simulink model "timeDelayedEKF_OOSM"  (R2015a)
settings: Solver=ode3  StartTime=0.0  StopTime=50  FixedStep=0.001  RelTol=1e-3
model workspace (MAT data in the model file):
  x_k = Simulink.Signal
  x_k.DataType = 'double'
  x_k.Dimensions = [2 1]
  x_k.DimensionsMode = 'Fixed'
  x_k.Complexity = 'real'
  x_k.SampleTime = -1
  x_k.SamplingMode = 'auto'
  x_k.InitialValue = '[0;0]'
  P_k = Simulink.Signal
  P_k.DataType = 'double'
  P_k.Dimensions = [2 2]
  P_k.DimensionsMode = 'Fixed'
  P_k.Complexity = 'real'
  P_k.SampleTime = -1
  P_k.SamplingMode = 'auto'
  P_k.InitialValue = '10*ones(2,2)'
  R = Simulink.Parameter
  R.Value = 0.001
  R.DataType = 'auto'
  t_delta = Simulink.Parameter
  t_delta.Value = 0.01
  t_delta.DataType = 'auto'
  x_d = Simulink.Signal
  x_d.DataType = 'auto'
  x_d.Dimensions = [2 1]
  x_d.DimensionsMode = 'auto'
  x_d.Complexity = 'auto'
  x_d.SampleTime = -1
  x_d.SamplingMode = 'auto'
  x_d.InitialValue = '[0;0]'
  P_d = Simulink.Signal
  P_d.DataType = 'auto'
  P_d.Dimensions = [2 2]
  P_d.DimensionsMode = 'auto'
  P_d.Complexity = 'auto'
  P_d.SampleTime = -1
  P_d.SamplingMode = 'auto'
  P_d.InitialValue = '10*eye(2,2)'
  U_n_d = Simulink.Signal
  U_n_d.DataType = 'auto'
  U_n_d.Dimensions = [2 2]
  U_n_d.DimensionsMode = 'auto'
  U_n_d.Complexity = 'auto'
  U_n_d.SampleTime = -1
  U_n_d.SamplingMode = 'auto'
  U_n_d.InitialValue = '10*eye(2,2)'
  FIFO_update_count = Simulink.Signal
  FIFO_update_count.DataType = 'auto'
  FIFO_update_count.Dimensions = -1
  FIFO_update_count.DimensionsMode = 'auto'
  FIFO_update_count.Complexity = 'auto'
  FIFO_update_count.SampleTime = -1
  FIFO_update_count.SamplingMode = 'auto'
  FIFO_update_count.InitialValue = '0'
  flag_OOSM_update = Simulink.Signal
  flag_OOSM_update.DataType = 'boolean'
  flag_OOSM_update.Dimensions = 1
  flag_OOSM_update.DimensionsMode = 'auto'
  flag_OOSM_update.Complexity = 'auto'
  flag_OOSM_update.SampleTime = -1
  flag_OOSM_update.SamplingMode = 'auto'
  flag_OOSM_update.InitialValue = 'false'
undefined symbols (not defined in the file): des, gcbh
libraries: simulink x5
settings Model: PauseTimes=0  NumberOfSteps=10  CovSFcnEnable=off  Creator=Iseberg  LastModifiedBy=Ana
settings DebuggingCC: SolverPrmCheckMsg=warning  MultiTaskDSMMsg=warning  MultiTaskCondExecSysMsg=warning  MultiTaskRateTransMsg=warning

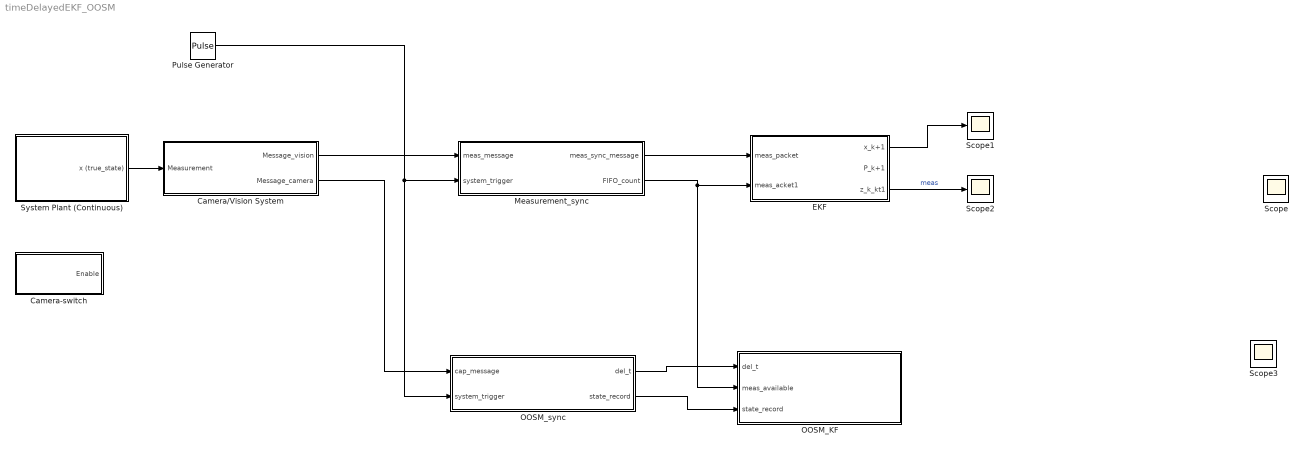
== system timeDelayedEKF_OOSM ==
  Camera-switch : Subsystem
  Camera/Vision System : Subsystem
  EKF : Subsystem
  Measurement_sync : Subsystem
  OOSM_KF : Subsystem
  OOSM_sync : Subsystem
  Pulse Generator : DiscretePulseGenerator  Period=10  SampleTime=0.001
  Scope{,1..3} (4 alike) : Scope
      Scope settings: YMin=0  YMax=1
      Scope1 settings: YMin=0  YMax=21000  SaveName=ScopeData12
      Scope2 settings: YMin=0  YMax=21000  SaveName=ScopeData3
      Scope3 settings: YMin=0  YMax=1  SaveName=ScopeData4
  System Plant (Continuous) : Subsystem
  wires:
  System Plant (Continuous)/1(x (true_state)) -> Camera/Vision System/1(Measurement)
  Camera/Vision System/1("Message_vision ") -> Measurement_sync/1(meas_message)
  Camera/Vision System/2("Message_camera ") -> OOSM_sync/1(cap_message)
  Pulse Generator/1 -> Measurement_sync/2("system_trigger "), OOSM_sync/2("system_trigger ")
  Measurement_sync/2(FIFO_count) -> EKF/2(meas_acket1), OOSM_KF/2(meas_available)
  OOSM_sync/1(del_t) -> OOSM_KF/1(del_t)
  Measurement_sync/1(meas_sync_message) -> EKF/1(meas_packet)
  EKF/3(z_k_kt1) -> Scope2/1  "meas"
  EKF/1(x_k+1) -> Scope1/1
  OOSM_sync/2(state_record) -> OOSM_KF/3("state_record ")

== system timeDelayedEKF_OOSM/Camera-switch ==
  Manual Switch : ManualSwitch
  Manual Switch1 : ManualSwitch  CurrentSetting=0
  Manual Switch2 : ManualSwitch
  Off_manual : Constant  Value=inf
  On_manual : Constant  Value=0.1
  Scope : Scope
      settings: SaveName=ScopeData6
  Step : Step  Time=abs(0.1*randn(1))  After=0.1  SampleTime=0
  intergeneration time : Constant  Value=0.1
  Enable : Outport
  wires:
  intergeneration time/1 -> Manual Switch/2
  Manual Switch2/1 -> Manual Switch1/1
  Off_manual/1 -> Manual Switch2/1
  Manual Switch1/1 -> Enable/1
  Step/1 -> Scope/1, Manual Switch/1
  Manual Switch/1 -> Manual Switch1/2
  On_manual/1 -> Manual Switch2/2

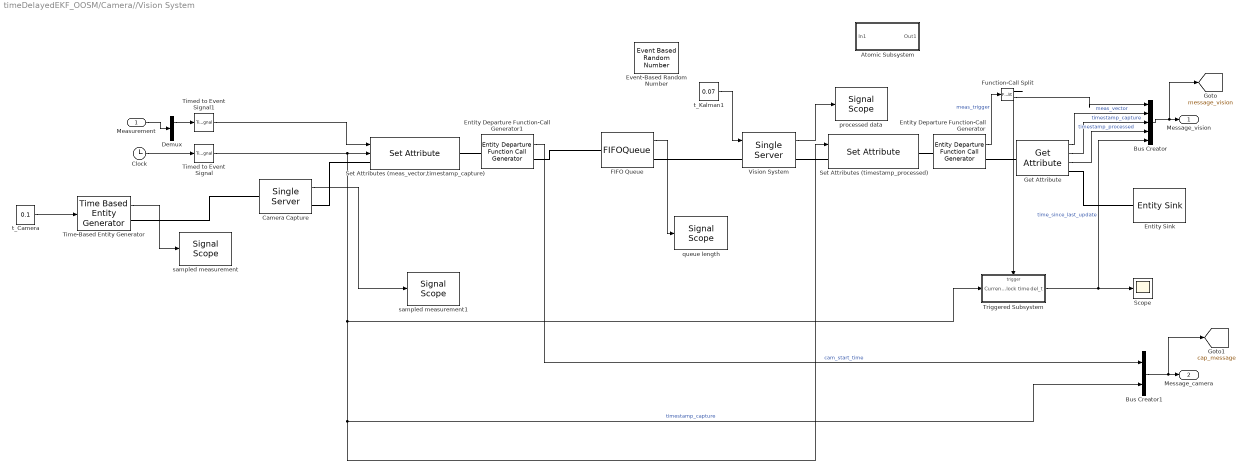
== system timeDelayedEKF_OOSM/Camera//Vision System ==
  Measurement : Inport
  Atomic Subsystem : Subsystem
  Bus Creator : BusCreator  Inputs=5
  Bus Creator1 : BusCreator  Inputs=2
  Camera Capture : SingleServer  ServiceTime=0  StatNumberDeparted=on
  Clock : Clock
      settings: Decimation=2
  Demux : Demux  Outputs=2
  Entity Departure Function-Call Generator : EntityDepartureFunctionCallGenerator
  Entity Departure Function-Call Generator1 : EntityDepartureFunctionCallGenerator  TimingFunctionCallF1=Before entity departure
  Entity Sink : EntitySink
  Event-Based Random Number : EventBasedRandomNumber  Distribution=Uniform  minUnif=0.05  maxUnif=0.08
  FIFO Queue : FIFOQueue  Capacity=1  StatNumberInBlock=on
      settings: OutputPortMap=o1
  Function-Call Split : FunctionCallSplit
  Get Attribute : GetAttribute  AttributeName=meas_vector|timestamp_capture|timestamp_processed  AttributeMissing=Error|Error|Error  AttributeDefaultValue=1|1|1  AttributeTreatAsVector=1|1|1  AttributeSendTiming=After entity departure|After entity departure|After entity departure  EvaluatedDefaultAttributeValue={ [];[];[]}
      settings: OutputPortMap=o1,o2,o3
  Scope : Scope
  Set Attributes (meas_vector,timestamp_capture) : SetAttribute  AttributeName=meas_vector|timestamp_capture  AttributeFrom=Signal port|Signal port  AttributeValue=1|1  AttributeTreatAsVector=1|1  EvaluatedAttributeValue={ [];[]}
      settings: InputPortMap=u0,u1
  Set Attributes (timestamp_processed) : SetAttribute  AttributeName=timestamp_processed  AttributeFrom=Signal port  EvaluatedAttributeValue={ []}
  Time-Based Entity Generator : TimeBasedEntityGenerator  GenerateEntitiesUpon=Intergeneration time from port t  StatNumberDeparted=on
  Timed to Event Signal : TimedToEventSignal
  Timed to Event Signal1 : TimedToEventSignal
  Triggered Subsystem : Subsystem  TreatAsAtomicUnit=on
  "Vision System " : SingleServer  ServiceTimeFrom=Signal port t  StatNumberDeparted=on
  processed data : SignalScope  LoadFcn=des.scope.CallbackSupport('seLoadFcn',gcbh)  StartFcn=des.scope.CallbackSupport('seStartFcn',gcbh)  StopFcn=des.scope.CallbackSupport('seStopFcn',gcbh)
      settings: CopyFcn=des.scope.CallbackSupport('seCopyFcn',gcbh)  DeleteFcn=des.scope.CallbackSupport('seDeleteFcn',gcbh)  PreSaveFcn=des.scope.CallbackSupport('sePreSaveFcn',gcbh)  NameChangeFcn=des.scope.CallbackSupport('seNameChangeFcn',gcbh)  OpenFcn=des.scope.CallbackSupport('seOpenFcn',gcbh)
  queue length : SignalScope  LoadFcn=des.scope.CallbackSupport('seLoadFcn',gcbh)  StartFcn=des.scope.CallbackSupport('seStartFcn',gcbh)  StopFcn=des.scope.CallbackSupport('seStopFcn',gcbh)
      settings: CopyFcn=des.scope.CallbackSupport('seCopyFcn',gcbh)  DeleteFcn=des.scope.CallbackSupport('seDeleteFcn',gcbh)  PreSaveFcn=des.scope.CallbackSupport('sePreSaveFcn',gcbh)  NameChangeFcn=des.scope.CallbackSupport('seNameChangeFcn',gcbh)  OpenFcn=des.scope.CallbackSupport('seOpenFcn',gcbh)
  sampled measurement : SignalScope  LoadFcn=des.scope.CallbackSupport('seLoadFcn',gcbh)  StartFcn=des.scope.CallbackSupport('seStartFcn',gcbh)  StopFcn=des.scope.CallbackSupport('seStopFcn',gcbh)
      settings: CopyFcn=des.scope.CallbackSupport('seCopyFcn',gcbh)  DeleteFcn=des.scope.CallbackSupport('seDeleteFcn',gcbh)  PreSaveFcn=des.scope.CallbackSupport('sePreSaveFcn',gcbh)  NameChangeFcn=des.scope.CallbackSupport('seNameChangeFcn',gcbh)  OpenFcn=des.scope.CallbackSupport('seOpenFcn',gcbh)
  sampled measurement1 : SignalScope  LoadFcn=des.scope.CallbackSupport('seLoadFcn',gcbh)  StartFcn=des.scope.CallbackSupport('seStartFcn',gcbh)  StopFcn=des.scope.CallbackSupport('seStopFcn',gcbh)
      settings: CopyFcn=des.scope.CallbackSupport('seCopyFcn',gcbh)  DeleteFcn=des.scope.CallbackSupport('seDeleteFcn',gcbh)  PreSaveFcn=des.scope.CallbackSupport('sePreSaveFcn',gcbh)  NameChangeFcn=des.scope.CallbackSupport('seNameChangeFcn',gcbh)  OpenFcn=des.scope.CallbackSupport('seOpenFcn',gcbh)
  t_Camera : Constant  Value=0.1
  t_Kalman1 : Constant  Value=0.07
  "Message_vision " : Outport
  "Message_camera " : Outport  Port=2
  tag scope: cap_message=global, message_vision=global
  wires:
  Timed to Event Signal1/1 -> Set Attributes (meas_vector,timestamp_capture)/1
  Timed to Event Signal/1 -> Triggered Subsystem/1(Current Clock time), Bus Creator1/2, Set Attributes (timestamp_processed)/1, Set Attributes (meas_vector,timestamp_capture)/2  "timestamp_capture"
  Get Attribute/3 -> Bus Creator/4  "timestamp_processed"
  Time-Based Entity Generator/1 -> sampled measurement/1
  FIFO Queue/1 -> queue length/1
  "Vision System "/1 -> processed data/1
  Entity Departure Function-Call Generator/1 -> Function-Call Split/1  "meas_trigger"
  Get Attribute/2 -> Bus Creator/3  "timestamp_capture"
  Get Attribute/1 -> Bus Creator/2  "meas_vector"
  Clock/1 -> Timed to Event Signal/1
  Triggered Subsystem/1(del_t) -> Bus Creator/5, Scope/1  "time_since_last_update"
  Bus Creator1/1 -> [cap_message], "Message_camera "/1
  Entity Departure Function-Call Generator1/1 -> Bus Creator1/1  "cam_start_time"
  t_Camera/1 -> Time-Based Entity Generator/1
  Camera Capture/1 -> sampled measurement1/1
  Function-Call Split/2 -> Bus Creator/1
  Function-Call Split/1 -> Triggered Subsystem/Trigger
  Measurement/1 -> Demux/1
  Demux/1 -> Timed to Event Signal1/1
  t_Kalman1/1 -> "Vision System "/1
  Bus Creator/1 -> [message_vision], "Message_vision "/1
  connections:
  Entity Departure Function-Call Generator/LConn1 -- Set Attributes (timestamp_processed)/RConn1
  Get Attribute/RConn1 -- Entity Sink/LConn1
  "Vision System "/RConn1 -- Set Attributes (timestamp_processed)/LConn1
  Get Attribute/LConn1 -- Entity Departure Function-Call Generator/RConn1
  Entity Departure Function-Call Generator1/RConn1 -- FIFO Queue/LConn1
  Set Attributes (meas_vector,timestamp_capture)/RConn1 -- Entity Departure Function-Call Generator1/LConn1
  FIFO Queue/RConn1 -- "Vision System "/LConn1
  Camera Capture/LConn1 -- Time-Based Entity Generator/RConn1
  Camera Capture/RConn1 -- Set Attributes (meas_vector,timestamp_capture)/LConn1

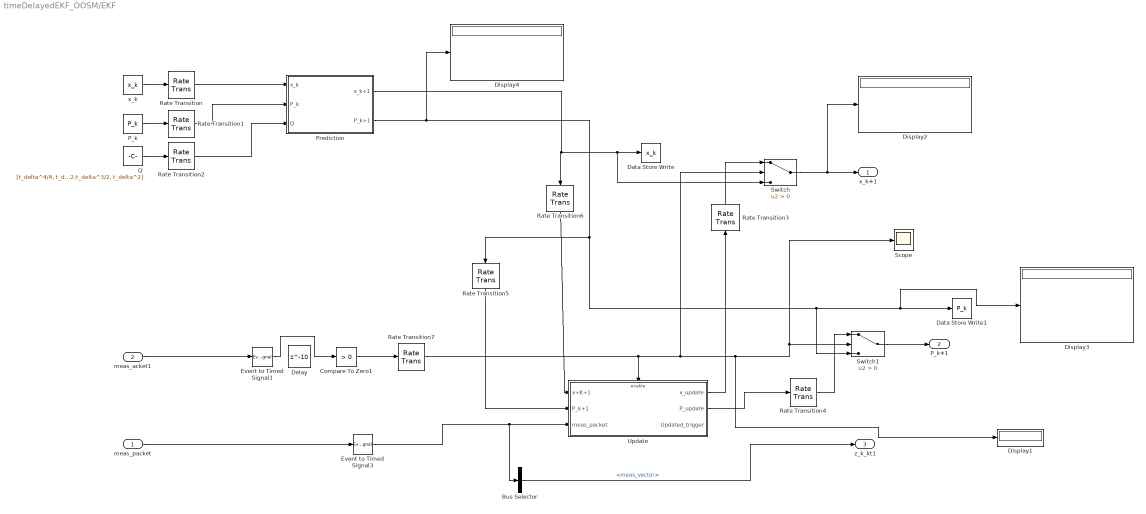
== system timeDelayedEKF_OOSM/EKF ==
  meas_packet : Inport
  meas_acket1 : Inport  Port=2
  Bus Selector : BusSelector  OutputSignals=meas_vector
  Compare To Zero1 : simulink/Logic and Bit Operations/Compare To Zero  relop=>  OutDataTypeStr=boolean
  Data Store Write : DataStoreWrite  DataStoreName=x_k  DataStoreElements=x_k
  Data Store Write1 : DataStoreWrite  DataStoreName=P_k  DataStoreElements=P_k
  Delay : Delay  DelayLength=10  InitialCondition=0
  Display{1..4} (4 alike) : Display
  Event to Timed Signal1 : EventToTimedSignal
  Event to Timed Signal3 : EventToTimedSignal
  P_k : DataStoreRead  DataStoreName=P_k  DataStoreElements=P_k
  Prediction : Subsystem  TreatAsAtomicUnit=on  SystemSampleTime=0.01
  Q : Constant  Value=[t_delta^4/4, t_delta^3/2;t_delta^3/2, t_delta^2]
  Rate Transition{,1..6} (7 alike) : RateTransition
  Rate Transition7 : RateTransition  OutPortSampleTime=0.01
  Scope : Scope
      settings: SaveName=ScopeData9
  Switch : Switch  Criteria=u2 > Threshold
  Switch1 : Switch  Criteria=u2 > Threshold
  Update : Subsystem  TreatAsAtomicUnit=on
  x_k : DataStoreRead  DataStoreName=x_k  DataStoreElements=x_k
  x_k+1 : Outport
  "P_k+1 " : Outport  Port=2
  z_k_kt1 : Outport  Port=3
  wires:
  x_k/1 -> Rate Transition/1
  P_k/1 -> Rate Transition1/1
  Q/1 -> Rate Transition2/1
  Prediction/1(x_k+1) -> Switch/3, Data Store Write/1, Rate Transition6/1
  Switch/1 -> Display2/1, x_k+1/1
  Switch1/1 -> "P_k+1 "/1
  Rate Transition/1 -> Prediction/1(x_k)
  Rate Transition1/1 -> Prediction/2(P_k)
  Rate Transition2/1 -> Prediction/3(Q)
  Prediction/2(P_k+1) -> Display4/1, Switch1/3, Display3/1, Data Store Write1/1, Rate Transition5/1
  Rate Transition6/1 -> Update/1(x+K+1)
  Rate Transition5/1 -> Update/2(P_k+1)
  Update/1(x_update) -> Rate Transition3/1
  Rate Transition4/1 -> Switch1/1
  Rate Transition3/1 -> Switch/1
  Update/2(P_update) -> Rate Transition4/1
  meas_packet/1 -> Event to Timed Signal3/1
  meas_acket1/1 -> Event to Timed Signal1/1
  Event to Timed Signal3/1 -> Bus Selector/1, Update/3(meas_packet)
  Rate Transition7/1 -> Switch/2, Display1/1, Scope/1, Switch1/2, Update/Enable
  Compare To Zero1/1 -> Rate Transition7/1
  Event to Timed Signal1/1 -> Compare To Zero1/1
  Bus Selector/1 -> z_k_kt1/1  "<meas_vector>"

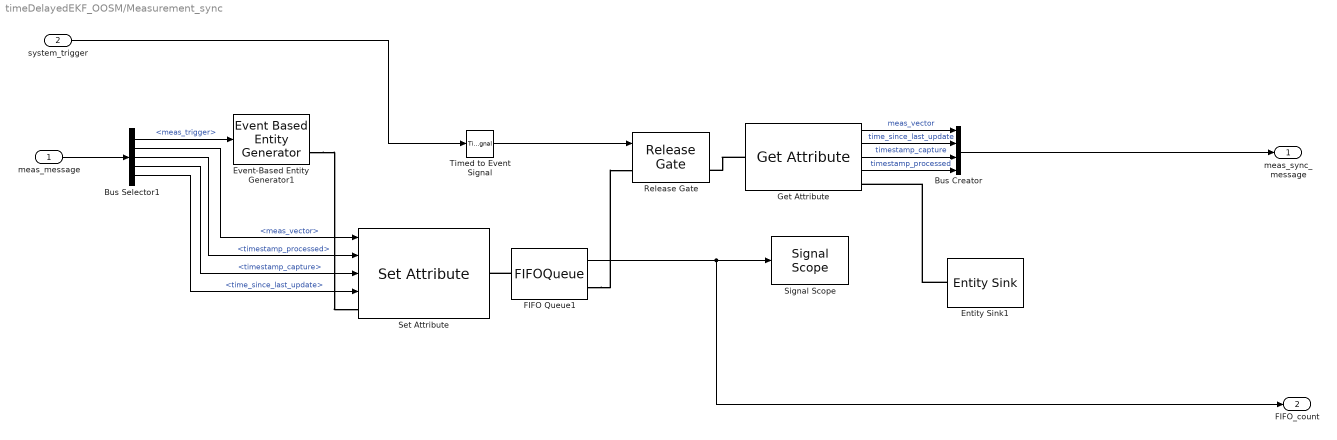
== system timeDelayedEKF_OOSM/Measurement_sync ==
  meas_message : Inport
  "system_trigger " : Inport  Port=2
  Bus Creator : BusCreator
  Bus Selector1 : BusSelector  OutputSignals=meas_trigger,meas_vector,timestamp_processed,timestamp_capture,time_since_last_update
  Entity Sink1 : EntitySink
  Event-Based Entity Generator1 : EventBasedEntityGenerator  GenerateEntitiesUpon=Function call from port fcn  StatNumberDeparted=on
  FIFO Queue1 : FIFOQueue  Capacity=1  StatNumberInBlock=on
      settings: OutputPortMap=o1
  Get Attribute : GetAttribute  AttributeName=meas_vector|time_since_last_update|timestamp_capture|timestamp_processed  AttributeMissing=Error|Error|Error|Error  AttributeDefaultValue=1|1|1|1  AttributeTreatAsVector=1|1|1|1  AttributeSendTiming=After entity departure|After entity departure|After entity departure|After entity departure  EvaluatedDefaultAttributeValue={ [];[];[];[]}
      settings: OutputPortMap=o1,o2,o3,o4
  Release Gate : ReleaseGate  StatNumberDeparted=on
  Set Attribute : SetAttribute  AttributeName=meas_vector|timestamp_processed|timestamp_capture|time_since_last_update  AttributeFrom=Signal port|Signal port|Signal port|Signal port  AttributeValue=1|1|1|1  AttributeTreatAsVector=1|1|1|1  EvaluatedAttributeValue={ [];[];[];[]}
      settings: InputPortMap=u0,u1,u2,u3
  Signal Scope : SignalScope  LoadFcn=des.scope.CallbackSupport('seLoadFcn',gcbh)  StartFcn=des.scope.CallbackSupport('seStartFcn',gcbh)  StopFcn=des.scope.CallbackSupport('seStopFcn',gcbh)
      settings: CopyFcn=des.scope.CallbackSupport('seCopyFcn',gcbh)  DeleteFcn=des.scope.CallbackSupport('seDeleteFcn',gcbh)  PreSaveFcn=des.scope.CallbackSupport('sePreSaveFcn',gcbh)  NameChangeFcn=des.scope.CallbackSupport('seNameChangeFcn',gcbh)  OpenFcn=des.scope.CallbackSupport('seOpenFcn',gcbh)
  Timed to Event Signal : TimedToEventSignal
  meas_sync_message : Outport
  FIFO_count : Outport  Port=2
  wires:
  Get Attribute/4 -> Bus Creator/4  "timestamp_processed"
  Bus Selector1/1 -> Event-Based Entity Generator1/1  "<meas_trigger>"
  Get Attribute/3 -> Bus Creator/3  "timestamp_capture"
  Bus Selector1/2 -> Set Attribute/1  "<meas_vector>"
  Get Attribute/2 -> Bus Creator/2  "time_since_last_update"
  "system_trigger "/1 -> Timed to Event Signal/1
  Get Attribute/1 -> Bus Creator/1  "meas_vector"
  Bus Selector1/5 -> Set Attribute/4  "<time_since_last_update>"
  Bus Selector1/3 -> Set Attribute/2  "<timestamp_processed>"
  Bus Selector1/4 -> Set Attribute/3  "<timestamp_capture>"
  Timed to Event Signal/1 -> Release Gate/1
  meas_message/1 -> Bus Selector1/1
  Bus Creator/1 -> meas_sync_message/1
  FIFO Queue1/1 -> FIFO_count/1, Signal Scope/1
  connections:
  Entity Sink1/LConn1 -- Get Attribute/RConn1
  FIFO Queue1/RConn1 -- Release Gate/LConn1
  Event-Based Entity Generator1/RConn1 -- Set Attribute/LConn1
  Get Attribute/LConn1 -- Release Gate/RConn1
  FIFO Queue1/LConn1 -- Set Attribute/RConn1

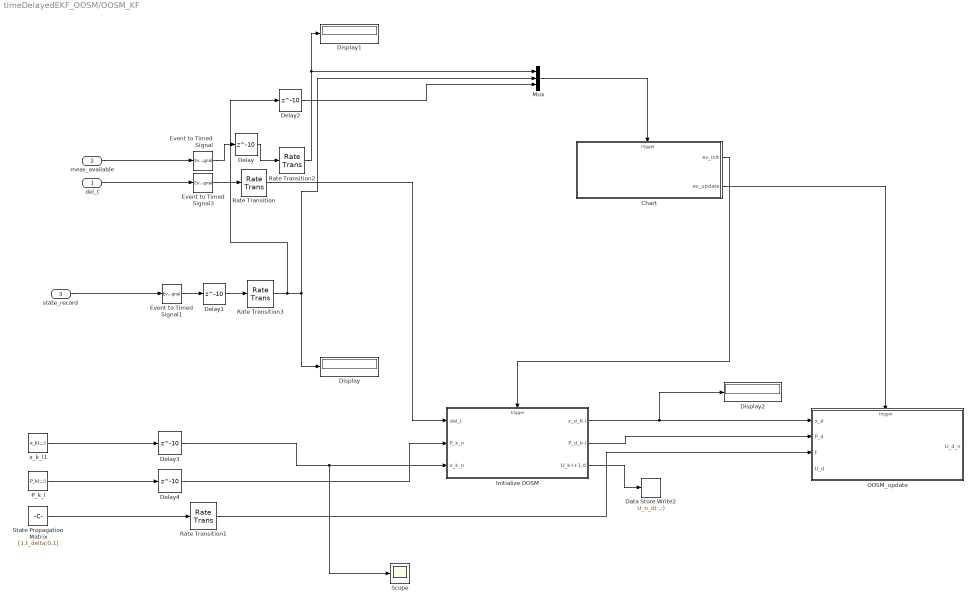
== system timeDelayedEKF_OOSM/OOSM_KF ==
  del_t : Inport
  meas_available : Inport  Port=2
  "state_record " : Inport  Port=3
  Chart : Stateflow chart  TreatAsAtomicUnit=on
  Data Store Write2 : DataStoreWrite  DataStoreName=U_n_d  DataStoreElements=U_n_d(:,:)
  Delay : Delay  DelayLength=10  InitialCondition=0
  Delay1 : Delay  DelayLength=10  InitialCondition=0
  Delay2 : Delay  DelayLength=10  InitialCondition=0
  Delay3 : Delay  DelayLength=10  InitialCondition=0  SampleTime=0.01
  Delay4 : Delay  DelayLength=10  InitialCondition=10  SampleTime=0.01
  Display : Display
  Display1 : Display
  Display2 : Display
  Event to Timed Signal : EventToTimedSignal
  Event to Timed Signal1 : EventToTimedSignal
  Event to Timed Signal3 : EventToTimedSignal
  Initialize OOSM : Subsystem  TreatAsAtomicUnit=on
  Mux : Mux  Inputs=3
  OOSM_update : Subsystem
  P_k_l : DataStoreRead  DataStoreName=P_k  DataStoreElements=P_k(:,:)
  Rate Transition{,1..3} (4 alike) : RateTransition
  Scope : Scope
      settings: SaveName=ScopeData14
  "State Propagation Matrix " : Constant  Value=[1,t_delta;0,1]
  x_k_l1 : DataStoreRead  DataStoreName=x_k  DataStoreElements=x_k(:,:)
  wires:
  "State Propagation Matrix "/1 -> Rate Transition1/1
  del_t/1 -> Event to Timed Signal3/1
  Event to Timed Signal3/1 -> Rate Transition/1
  meas_available/1 -> Event to Timed Signal/1
  Event to Timed Signal1/1 -> Delay1/1
  Delay1/1 -> Rate Transition3/1
  "state_record "/1 -> Event to Timed Signal1/1
  Rate Transition3/1 -> Delay2/1, Mux/2, Display/1
  Event to Timed Signal/1 -> Delay/1
  Rate Transition2/1 -> Mux/1, Display1/1
  P_k_l/1 -> Delay4/1
  x_k_l1/1 -> Delay3/1
  Delay4/1 -> Initialize OOSM/2(P_k_n)
  Delay3/1 -> Scope/1, Initialize OOSM/3(x_k_n)
  Rate Transition/1 -> Initialize OOSM/1(del_t)
  Initialize OOSM/1(x_d_K-l) -> Display2/1, OOSM_update/1(x_d)
  Initialize OOSM/2(P_d_k-l) -> OOSM_update/2(P_d)
  Rate Transition1/1 -> OOSM_update/3(F)
  Mux/1 -> Chart/Trigger
  Chart/1(ev_init) -> Initialize OOSM/Trigger
  Chart/2(ev_update) -> OOSM_update/Trigger
  Delay/1 -> Rate Transition2/1
  Delay2/1 -> Mux/3
  Initialize OOSM/3(U_k-l+1,d) -> Data Store Write2/1

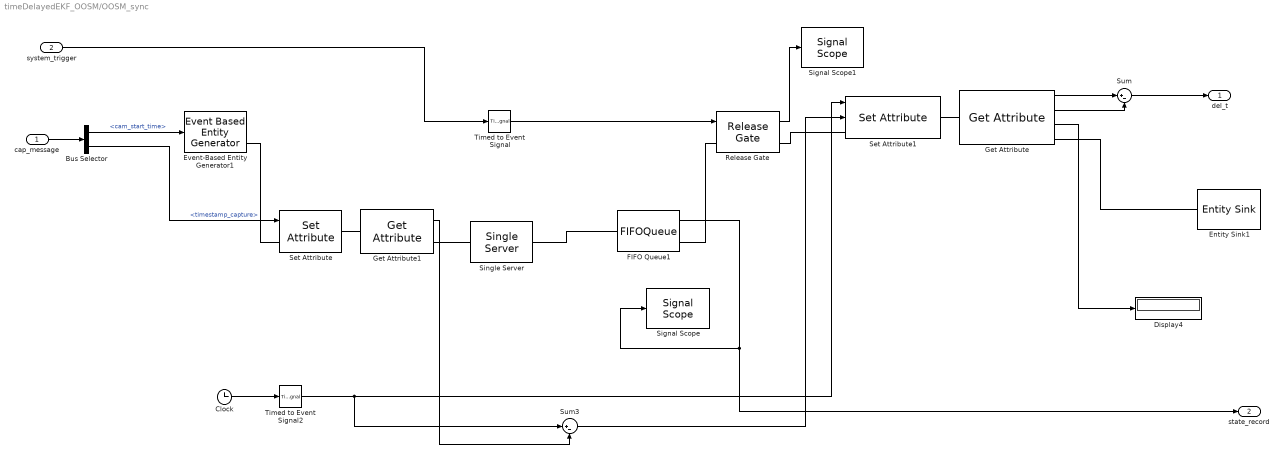
== system timeDelayedEKF_OOSM/OOSM_sync ==
  cap_message : Inport
  "system_trigger " : Inport  Port=2
  Bus Selector : BusSelector  OutputSignals=cam_start_time,timestamp_capture
  Clock : Clock
  Display4 : Display
  Entity Sink1 : EntitySink
  Event-Based Entity Generator1 : EventBasedEntityGenerator  GenerateEntitiesUpon=Function call from port fcn  StatNumberDeparted=on
  FIFO Queue1 : FIFOQueue  Capacity=5  StatNumberInBlock=on
      settings: OutputPortMap=o1
  Get Attribute : GetAttribute  AttributeName=timestamp_KFTrigger|timestamp_capture|t_delta_oosm  AttributeMissing=Error|Error|Error  AttributeDefaultValue=1|1|1  AttributeTreatAsVector=1|1|1  AttributeSendTiming=After entity departure|After entity departure|After entity departure  EvaluatedDefaultAttributeValue={ [];[];[]}
      settings: OutputPortMap=o1,o2,o3
  Get Attribute1 : GetAttribute  AttributeName=timestamp_capture  EvaluatedDefaultAttributeValue={ []}
      settings: OutputPortMap=o1
  Release Gate : ReleaseGate  StatNumberDeparted=on
  Set Attribute : SetAttribute  AttributeName=timestamp_capture  AttributeFrom=Signal port  EvaluatedAttributeValue={ []}
  Set Attribute1 : SetAttribute  AttributeName=timestamp_KFTrigger|t_delta_oosm  AttributeFrom=Signal port|Signal port  AttributeValue=1|1  AttributeTreatAsVector=1|1  EvaluatedAttributeValue={ [];[]}
      settings: InputPortMap=u0,u1
  Signal Scope : SignalScope  LoadFcn=des.scope.CallbackSupport('seLoadFcn',gcbh)  StartFcn=des.scope.CallbackSupport('seStartFcn',gcbh)  StopFcn=des.scope.CallbackSupport('seStopFcn',gcbh)
      settings: CopyFcn=des.scope.CallbackSupport('seCopyFcn',gcbh)  DeleteFcn=des.scope.CallbackSupport('seDeleteFcn',gcbh)  PreSaveFcn=des.scope.CallbackSupport('sePreSaveFcn',gcbh)  NameChangeFcn=des.scope.CallbackSupport('seNameChangeFcn',gcbh)  OpenFcn=des.scope.CallbackSupport('seOpenFcn',gcbh)
  Signal Scope1 : SignalScope  LoadFcn=des.scope.CallbackSupport('seLoadFcn',gcbh)  StartFcn=des.scope.CallbackSupport('seStartFcn',gcbh)  StopFcn=des.scope.CallbackSupport('seStopFcn',gcbh)
      settings: CopyFcn=des.scope.CallbackSupport('seCopyFcn',gcbh)  DeleteFcn=des.scope.CallbackSupport('seDeleteFcn',gcbh)  PreSaveFcn=des.scope.CallbackSupport('sePreSaveFcn',gcbh)  NameChangeFcn=des.scope.CallbackSupport('seNameChangeFcn',gcbh)  OpenFcn=des.scope.CallbackSupport('seOpenFcn',gcbh)
  Single Server : SingleServer  ServiceTime=0
  Sum : Sum  Inputs=|+-
  Sum3 : Sum  Inputs=|+-
  Timed to Event Signal : TimedToEventSignal
  Timed to Event Signal2 : TimedToEventSignal
  del_t : Outport
  state_record : Outport  Port=2
  wires:
  FIFO Queue1/1 -> state_record/1, Signal Scope/1
  Bus Selector/1 -> Event-Based Entity Generator1/1  "<cam_start_time>"
  Bus Selector/2 -> Set Attribute/1  "<timestamp_capture>"
  Clock/1 -> Timed to Event Signal2/1
  Timed to Event Signal2/1 -> Sum3/1, Set Attribute1/1
  Get Attribute/1 -> Sum/1
  Get Attribute/2 -> Sum/2
  Get Attribute1/1 -> Sum3/2
  Sum3/1 -> Set Attribute1/2
  cap_message/1 -> Bus Selector/1
  "system_trigger "/1 -> Timed to Event Signal/1
  Timed to Event Signal/1 -> Release Gate/1
  Get Attribute/3 -> Display4/1
  Release Gate/1 -> Signal Scope1/1
  Sum/1 -> del_t/1
  connections:
  Event-Based Entity Generator1/RConn1 -- Set Attribute/LConn1
  FIFO Queue1/RConn1 -- Release Gate/LConn1
  Release Gate/RConn1 -- Set Attribute1/LConn1
  Set Attribute1/RConn1 -- Get Attribute/LConn1
  Get Attribute1/LConn1 -- Set Attribute/RConn1
  Single Server/RConn1 -- FIFO Queue1/LConn1
  Get Attribute1/RConn1 -- Single Server/LConn1
  Entity Sink1/LConn1 -- Get Attribute/RConn1

== system timeDelayedEKF_OOSM/System Plant (Continuous) ==
  Integrator : Integrator  InitialConditionSource=external
  Product1 : Product  Multiplication=Matrix(*)
  State Matrix 1 : Constant  Value=[5;1]
  State Matrix 2 : Constant  Value=[0,1;0,0]
  x (true_state) : Outport
  wires:
  State Matrix 1/1 -> Integrator/2
  State Matrix 2/1 -> Product1/1
  Integrator/1 -> x (true_state)/1, Product1/2
  Product1/1 -> Integrator/1

== system timeDelayedEKF_OOSM/Camera//Vision System/Atomic Subsystem ==
  In1 : Inport
  Constant : Constant  Value=100
  Gain : Gain  Gain=100
  Product : Product
  Rounding Function : Rounding
  Scope : Scope
      settings: SaveName=ScopeData5
  Out1 : Outport
  wires:
  In1/1 -> Gain/1
  Gain/1 -> Rounding Function/1
  Constant/1 -> Product/2
  Product/1 -> Scope/1, Out1/1
  Rounding Function/1 -> Product/1

== system timeDelayedEKF_OOSM/Camera//Vision System/Triggered Subsystem ==
  Current Clock time : Inport
  Trigger : TriggerPort  TriggerType=function-call
  Delay : Delay  DelayLength=1  InitialCondition=0
  Sum : Sum  Inputs=|+-
  del_t : Outport
  wires:
  Current Clock time/1 -> Sum/1, Delay/1
  Sum/1 -> del_t/1
  Delay/1 -> Sum/2

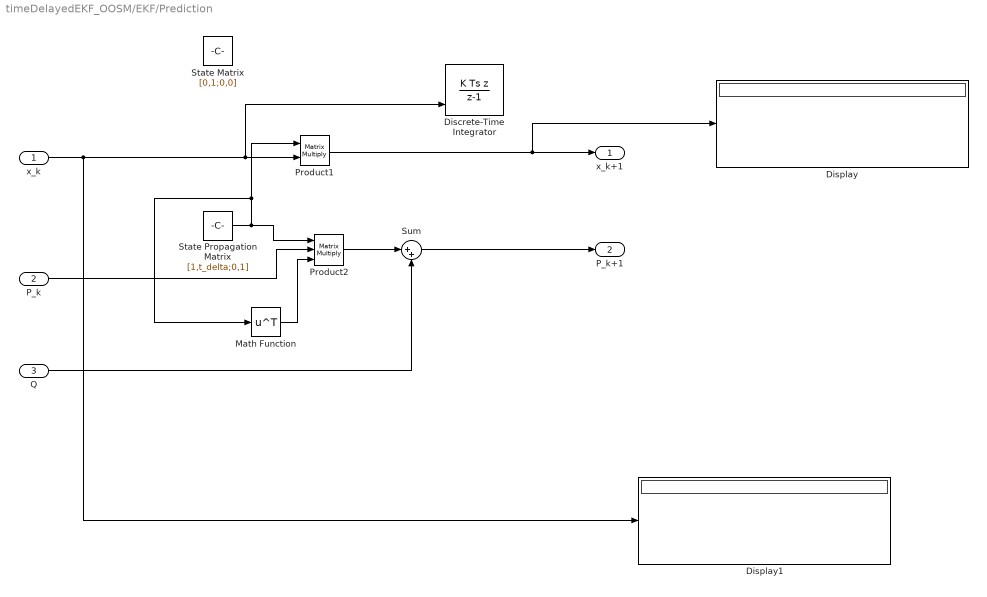
== system timeDelayedEKF_OOSM/EKF/Prediction ==
  x_k : Inport
  P_k : Inport  Port=2
  Q : Inport  Port=3
  Discrete-Time Integrator : DiscreteIntegrator  IntegratorMethod=Integration: Backward Euler  ExternalReset=rising  InitialConditionSource=external  InitialCondition=x_k  SampleTime=-1
  Display : Display
  Display1 : Display
  Math Function : Math  Operator=transpose  SaturateOnIntegerOverflow=on
  Product1 : Product  Multiplication=Matrix(*)
  Product2 : Product  Inputs=3  Multiplication=Matrix(*)
  State Matrix : Constant  Value=[0,1;0,0]
  "State Propagation Matrix " : Constant  Value=[1,t_delta;0,1]
  Sum : Sum  Inputs=|++
  x_k+1 : Outport
  P_k+1 : Outport  Port=2
  wires:
  Product2/1 -> Sum/1
  Q/1 -> Sum/2
  P_k/1 -> Product2/2
  Sum/1 -> P_k+1/1
  "State Propagation Matrix "/1 -> Product1/1, Math Function/1, Product2/1
  Math Function/1 -> Product2/3
  x_k/1 -> Display1/1, Discrete-Time Integrator/3, Product1/2
  Product1/1 -> Display/1, x_k+1/1

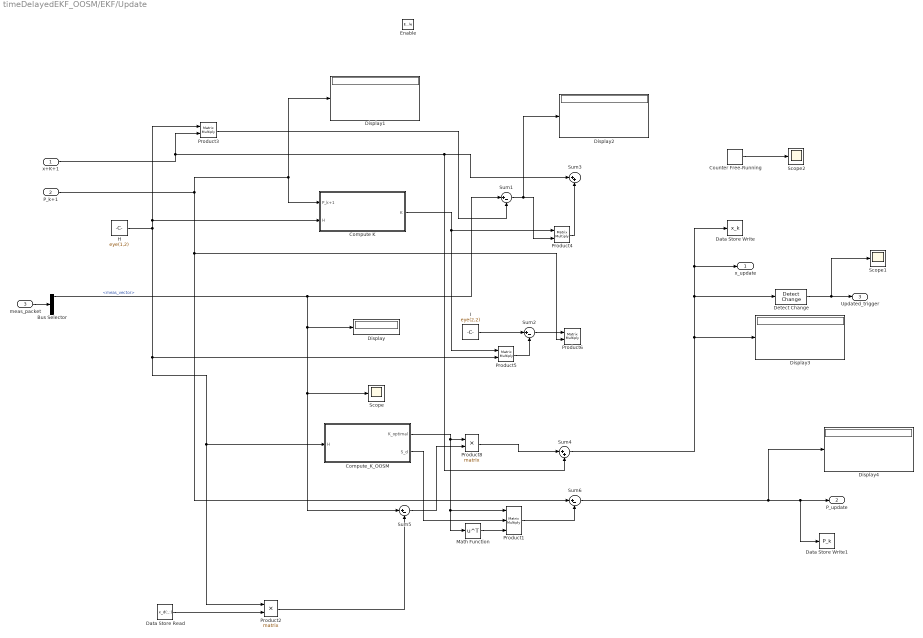
== system timeDelayedEKF_OOSM/EKF/Update ==
  x+K+1 : Inport
  P_k+1 : Inport  Port=2
  meas_packet : Inport  Port=3
  Enable : EnablePort
  Bus Selector : BusSelector  OutputSignals=meas_vector,time_since_last_update,timestamp_capture,timestamp_processed
  Compute K : Subsystem
  Compute_K_OOSM : Subsystem
  Counter Free-Running : simulink/Sources/Counter Free-Running  NumBits=16  tsamp=-1
  Data Store Read : DataStoreRead  DataStoreName=x_d  DataStoreElements=x_d(:,:)
  Data Store Write : DataStoreWrite  DataStoreName=x_k
  Data Store Write1 : DataStoreWrite  DataStoreName=P_k
  Detect Change : simulink/Logic and Bit Operations/Detect Change  vinit=0  InputProcessing=Inherited  OutDataTypeStr=boolean
  Display{,1..4} (5 alike) : Display
  H : Constant  Value=eye(1,2)  VectorParams1D=off
  I : Constant  Value=eye(2,2)
  Math Function : Math  Operator=transpose  SaturateOnIntegerOverflow=on
  Product1 : Product  Inputs=3  Multiplication=Matrix(*)
  Product{2..6,8} (6 alike) : Product  Multiplication=Matrix(*)
  Scope : Scope
      settings: TimeRange=5  SaveName=ScopeData11
  Scope1 : Scope
      settings: TimeRange=5  SaveName=ScopeData7
  Scope2 : Scope
      settings: TimeRange=50  YMin=0  YMax=4  SaveName=ScopeData8
  Sum{1..2,5..6} (4 alike) : Sum  Inputs=|+-
  Sum3 : Sum  Inputs=|++
  Sum4 : Sum  Inputs=|++
  x_update : Outport
  P_update : Outport  Port=2
  Updated_trigger : Outport  Port=3
  wires:
  P_k+1/1 -> Compute K/1(P_k+1), Display1/1, Sum6/1, Product6/2
  H/1 -> Compute K/2(H), Product3/1, Product2/1, Compute_K_OOSM/1(H), Product5/2
  x+K+1/1 -> Sum4/2, Sum3/1, Product3/2
  Bus Selector/1 -> Sum1/1, Display/1, Scope/1, Sum5/1  "<meas_vector>"
  Product3/1 -> Sum1/2
  Sum1/1 -> Display2/1, Product4/2
  Product4/1 -> Sum3/2
  I/1 -> Sum2/1
  Product5/1 -> Sum2/2
  Sum2/1 -> Product6/1
  Sum6/1 -> Display4/1, Data Store Write1/1, P_update/1
  Sum4/1 -> Data Store Write/1, x_update/1, Detect Change/1, Display3/1
  Compute K/1(K) -> Product5/1, Product4/1
  Data Store Read/1 -> Product2/2
  Product2/1 -> Sum5/2
  Compute_K_OOSM/1(K_optimal) -> Product1/1, Math Function/1, Product8/1
  Sum5/1 -> Product8/2
  Product8/1 -> Sum4/1
  Compute_K_OOSM/2(S_d) -> Product1/2
  Math Function/1 -> Product1/3
  Product1/1 -> Sum6/2
  Detect Change/1 -> Scope1/1, Updated_trigger/1
  Counter Free-Running/1 -> Scope2/1
  meas_packet/1 -> Bus Selector/1

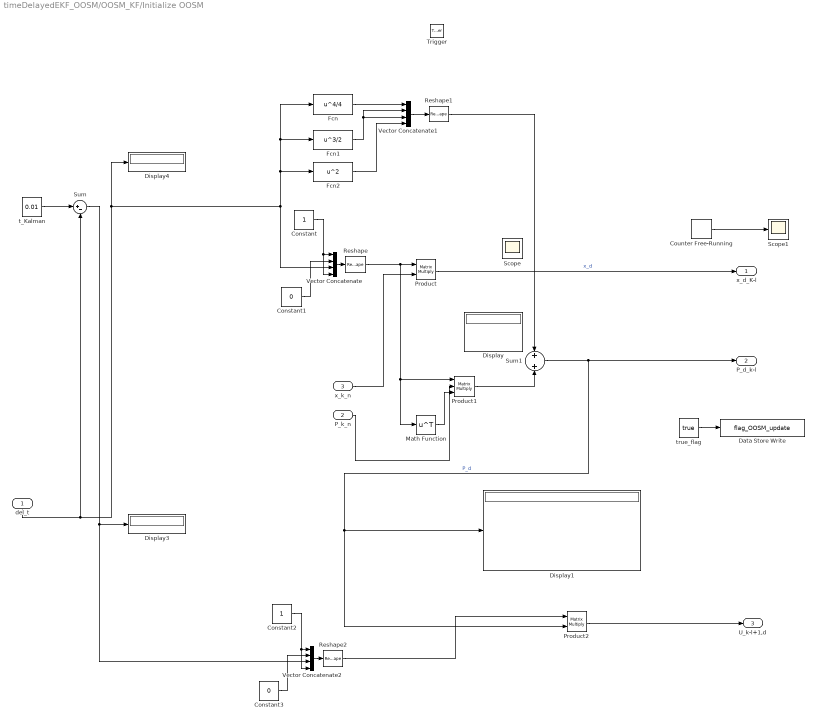
== system timeDelayedEKF_OOSM/OOSM_KF/Initialize OOSM ==
  del_t : Inport
  P_k_n : Inport  Port=2
  x_k_n : Inport  Port=3
  Trigger : TriggerPort  PortDimensions=1
  Constant : Constant
  Constant1 : Constant  Value=0
  Constant2 : Constant
  Constant3 : Constant  Value=0
  Counter Free-Running : simulink/Sources/Counter Free-Running  NumBits=16  tsamp=-1
  Data Store Write : DataStoreWrite  DataStoreName=flag_OOSM_update  DataStoreElements=flag_OOSM_update
  Display{,1,3..4} (4 alike) : Display
  Fcn : Fcn  Expr=u^4/4
  Fcn1 : Fcn  Expr=u^3/2
  Fcn2 : Fcn  Expr=u^2
  Math Function : Math  Operator=transpose  SaturateOnIntegerOverflow=on
  Product : Product  Multiplication=Matrix(*)
  Product1 : Product  Inputs=3  Multiplication=Matrix(*)
  Product2 : Product  Multiplication=Matrix(*)
  Reshape : Reshape  OutputDimensionality=Customize  OutputDimensions=[2,2]
  Reshape1 : Reshape  OutputDimensionality=Customize  OutputDimensions=[2,2]
  Reshape2 : Reshape  OutputDimensionality=Customize  OutputDimensions=[2,2]
  Scope : Scope
      settings: SaveName=ScopeData10
  Scope1 : Scope
      settings: SaveName=ScopeData2
  Sum : Sum  Inputs=|+-
  Sum1 : Sum
  Vector Concatenate : Concatenate  NumInputs=4
  Vector Concatenate1 : Concatenate  NumInputs=4
  Vector Concatenate2 : Concatenate  NumInputs=4
  t_Kalman : Constant  Value=0.01
  true_flag : Constant  Value=true
  x_d_K-l : Outport
  P_d_k-l : Outport  Port=2
  U_k-l+1,d : Outport  Port=3
  wires:
  Constant/1 -> Vector Concatenate/4, Vector Concatenate/1
  Constant1/1 -> Vector Concatenate/2
  Vector Concatenate/1 -> Reshape/1
  Math Function/1 -> Product1/3
  Fcn/1 -> Vector Concatenate1/1
  Fcn1/1 -> Vector Concatenate1/3, Vector Concatenate1/2
  Fcn2/1 -> Vector Concatenate1/4
  Vector Concatenate1/1 -> Reshape1/1
  Product1/1 -> Sum1/2
  Product/1 -> x_d_K-l/1  "x_d"
  Reshape1/1 -> Sum1/1
  Sum1/1 -> P_d_k-l/1, Product2/2, Display1/1  "P_d"
  Reshape/1 -> Product1/1, Math Function/1, Product/1
  Product2/1 -> U_k-l+1,d/1
  Constant2/1 -> Vector Concatenate2/4, Vector Concatenate2/1
  Constant3/1 -> Vector Concatenate2/2
  Vector Concatenate2/1 -> Reshape2/1
  Reshape2/1 -> Product2/1
  del_t/1 -> Fcn2/1, Fcn1/1, Fcn/1, Vector Concatenate/3, Display4/1, Sum/2
  t_Kalman/1 -> Sum/1
  true_flag/1 -> Data Store Write/1
  Counter Free-Running/1 -> Scope1/1
  Sum/1 -> Vector Concatenate2/3, Display3/1
  x_k_n/1 -> Product/2
  P_k_n/1 -> Product1/2

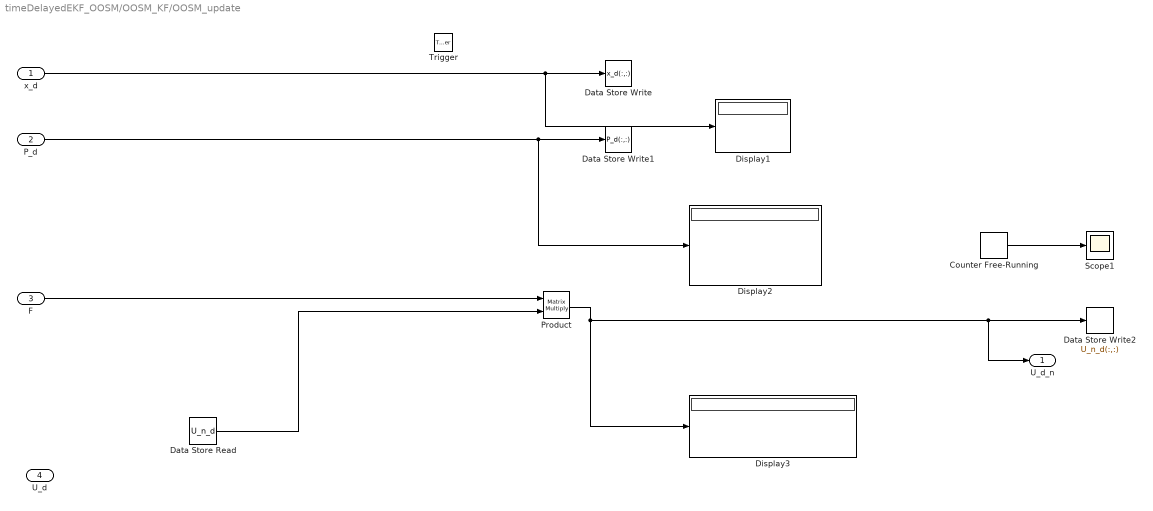
== system timeDelayedEKF_OOSM/OOSM_KF/OOSM_update ==
  x_d : Inport
  P_d : Inport  Port=2
  F : Inport  Port=3
  "U_d " : Inport  Port=4
  Trigger : TriggerPort  PortDimensions=1
  Counter Free-Running : simulink/Sources/Counter Free-Running  NumBits=16  tsamp=-1
  Data Store Read : DataStoreRead  DataStoreName=U_n_d
  Data Store Write : DataStoreWrite  DataStoreName=x_d  DataStoreElements=x_d(:,:)
  Data Store Write1 : DataStoreWrite  DataStoreName=P_d  DataStoreElements=P_d(:,:)
  Data Store Write2 : DataStoreWrite  DataStoreName=U_n_d  DataStoreElements=U_n_d(:,:)
  Display1 : Display
  Display2 : Display
  Display3 : Display
  Product : Product  Multiplication=Matrix(*)
  Scope1 : Scope
      settings: SaveName=ScopeData13
  U_d_n : Outport
  wires:
  x_d/1 -> Display1/1, Data Store Write/1
  P_d/1 -> Display2/1, Data Store Write1/1
  F/1 -> Product/1
  Data Store Read/1 -> Product/2
  Counter Free-Running/1 -> Scope1/1
  Product/1 -> Display3/1, U_d_n/1, Data Store Write2/1

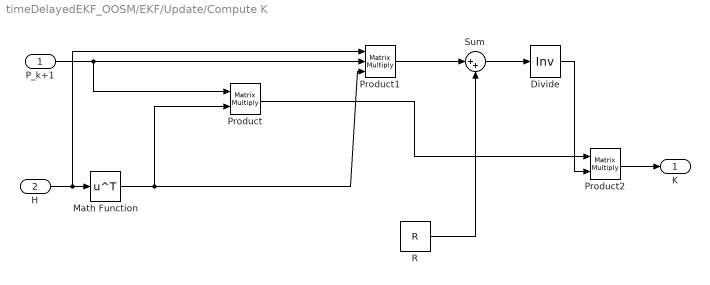
== system timeDelayedEKF_OOSM/EKF/Update/Compute K ==
  P_k+1 : Inport
  H : Inport  Port=2
  Divide : Product  Inputs=/  Multiplication=Matrix(*)
  Math Function : Math  Operator=transpose  SaturateOnIntegerOverflow=on
  Product : Product  Multiplication=Matrix(*)
  Product1 : Product  Inputs=3  Multiplication=Matrix(*)
  Product2 : Product  Multiplication=Matrix(*)
  R : Constant  Value=R
  Sum : Sum  Inputs=|++
  K : Outport
  wires:
  P_k+1/1 -> Product/1, Product1/2
  H/1 -> Product1/1, Math Function/1
  Sum/1 -> Divide/1
  Product1/1 -> Sum/1
  Divide/1 -> Product2/2
  Product2/1 -> K/1
  Product/1 -> Product2/1
  Math Function/1 -> Product/2, Product1/3
  R/1 -> Sum/2

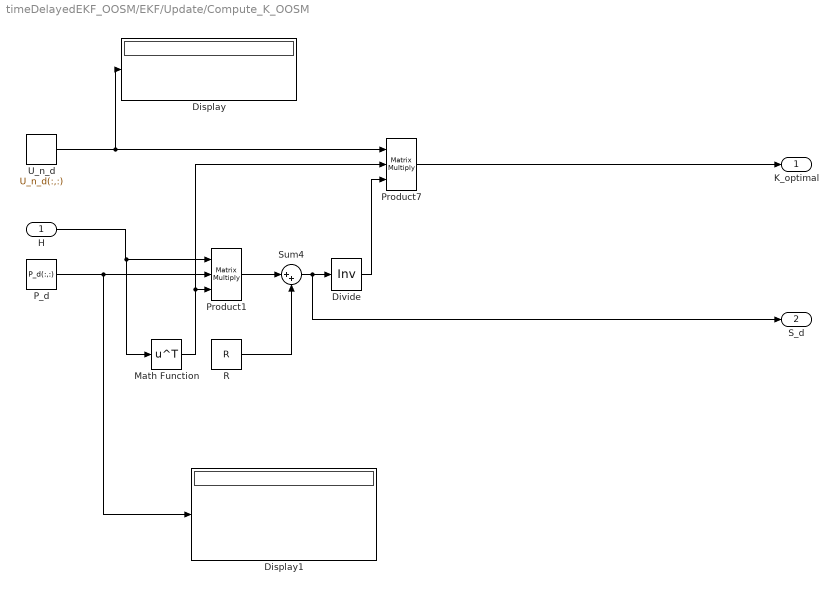
== system timeDelayedEKF_OOSM/EKF/Update/Compute_K_OOSM ==
  H : Inport
  Display : Display
  Display1 : Display
  Divide : Product  Inputs=/  Multiplication=Matrix(*)
  Math Function : Math  Operator=transpose  SaturateOnIntegerOverflow=on
  P_d : DataStoreRead  DataStoreName=P_d  DataStoreElements=P_d(:,:)
  Product1 : Product  Inputs=3  Multiplication=Matrix(*)
  Product7 : Product  Inputs=3  Multiplication=Matrix(*)
  R : Constant  Value=R
  Sum4 : Sum  Inputs=|++
  U_n_d : DataStoreRead  DataStoreName=U_n_d  DataStoreElements=U_n_d(:,:)
  K_optimal : Outport
  S_d : Outport  Port=2
  wires:
  Math Function/1 -> Product7/2, Product1/3
  R/1 -> Sum4/2
  U_n_d/1 -> Display/1, Product7/1
  P_d/1 -> Display1/1, Product1/2
  Product1/1 -> Sum4/1
  H/1 -> Math Function/1, Product1/1
  Product7/1 -> K_optimal/1
  Divide/1 -> Product7/3
  Sum4/1 -> S_d/1, Divide/1

== stateflow chart timeDelayedEKF_OOSM/OOSM_KF/Chart ==
  state state_foo/
    entry:
    state state_wait/
      entry:
    state state_update/
      bind:ev_update;
      entry:
      send(ev_update);
      during:
      send(ev_update);
    state state_init/
      bind:ev_init;
      entry:
      send(ev_init);
    (default) -> state_init
    state_update -> state_update [order 2]
    state_update -> state_wait [order 1] : meas_trigger
    state_init -> state_update : update
    state_wait -> state_init : record_state
  events: meas_trigger input RISING_EDGE_EVENT; record_state input RISING_EDGE_EVENT; ev_init output EITHER_EDGE_EVENT; ev_update output EITHER_EDGE_EVENT; update input RISING_EDGE_EVENT
